simulink model "test_3"  (R2022b)
settings: Solver=VariableStepAuto  StartTime=0.0  StopTime=120  RelTol=1e-3
undefined symbols (not defined in the file): c, DenPlant, NumPlant
settings Model: Creator=JOWAKO  LastModifiedBy=JOWAKO

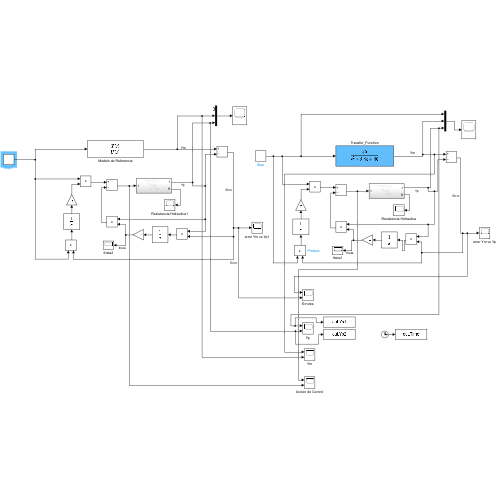
[thumbnail: Simulink's stored preview of the top-level diagram]
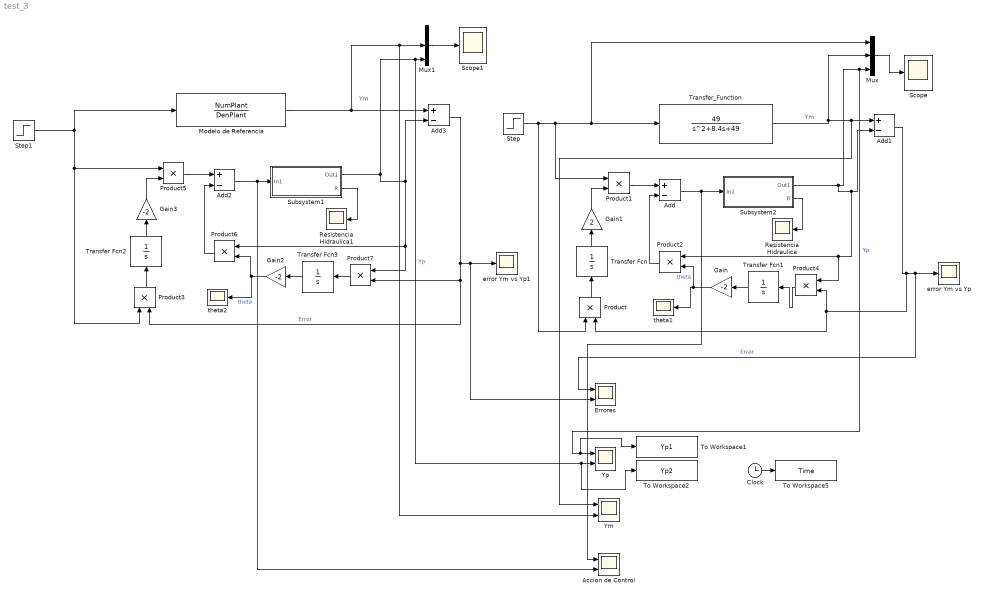
== system test_3 ==
  note: Ym
  note: Ym
  Accion de Control : Scope  NumInputPorts=2
  Add{,1..3} (4 alike) : Sum  Inputs=+-
  Clock : Clock
  Errores : Scope  NumInputPorts=2
  Gain : Gain  Gain=-2
  Gain1 : Gain  Gain=2
  Gain2 : Gain  Gain=-2
  Gain3 : Gain  Gain=-2
  Modelo de Referencia : TransferFcn  Numerator=NumPlant  Denominator=DenPlant
  Mux : Mux  Inputs=3
  Mux1 : Mux  Inputs=3
  Product{,1..7} (8 alike) : Product
  Resistencia Hidraulica : Scope
  Resistencia Hidraulica1 : Scope
  Scope : Scope
  Scope1 : Scope
  Step : Step  SampleTime=0
  Step1 : Step  SampleTime=0
  Subsystem1 : Subsystem
  Subsystem2 : Subsystem
  To Workspace1 : ToWorkspace  VariableName=Yp1  SaveFormat=Timeseries  SampleTime=-1
  To Workspace2 : ToWorkspace  VariableName=Yp2  SaveFormat=Timeseries  SampleTime=-1
  To Workspace5 : ToWorkspace  VariableName=Time  SaveFormat=Timeseries  SampleTime=-1
  Transfer Fcn{,1..3} (4 alike) : TransferFcn  Denominator=[1 0]
  Transfer_Function : TransferFcn  Numerator=49  Denominator=[1 8.4 49]
  Ym : Scope  NumInputPorts=2
  Yp : Scope  NumInputPorts=2
  error Ym vs Yp : Scope
  error Ym vs Yp1 : Scope
  theta1 : Scope
  theta2 : Scope
  wires:
  Subsystem2/2(R) -> Resistencia Hidraulica/1
  Transfer Fcn1/1 -> Gain/1
  Step1/1 -> Modelo de Referencia/1, Product5/1, Product3/1
  Transfer Fcn/1 -> Gain1/1
  Product2/1 -> Add/2
  Product1/1 -> Add/1
  Subsystem2/1(Out1) -> Add1/2, Product2/1, Product4/1, To Workspace1/1, Yp/1, Mux/3  "Yp"
  Add/1 -> Subsystem2/1(In1), Accion de Control/1
  Mux/1 -> Scope/1
  Gain1/1 -> Product1/2
  Transfer_Function/1 -> Mux/2, Ym/1, Add1/1
  Product/1 -> Transfer Fcn/1
  Add1/1 -> Errores/1, error Ym vs Yp/1, Product4/2, Product/2  "Error"
  Gain/1 -> theta1/1, Product2/2  "theta"
  Product4/1 -> Transfer Fcn1/1
  Subsystem1/2(R) -> Resistencia Hidraulica1/1
  Transfer Fcn3/1 -> Gain2/1
  Transfer Fcn2/1 -> Gain3/1
  Product6/1 -> Add2/2
  Product5/1 -> Add2/1
  Subsystem1/1(Out1) -> Add3/2, Product6/1, Product7/1, To Workspace2/1, Yp/2, Mux1/3  "Yp"
  Add2/1 -> Accion de Control/2, Subsystem1/1(In1)
  Mux1/1 -> Scope1/1
  Gain3/1 -> Product5/2
  Modelo de Referencia/1 -> Ym/2, Mux1/2, Add3/1
  Product3/1 -> Transfer Fcn2/1
  Add3/1 -> error Ym vs Yp1/1, Errores/2, Product3/2, Product7/2  "Error"
  Gain2/1 -> theta2/1, Product6/2  "theta"
  Product7/1 -> Transfer Fcn3/1
  Clock/1 -> To Workspace5/1
  Step/1 -> Product/1, Product1/1, Mux/1, Transfer_Function/1

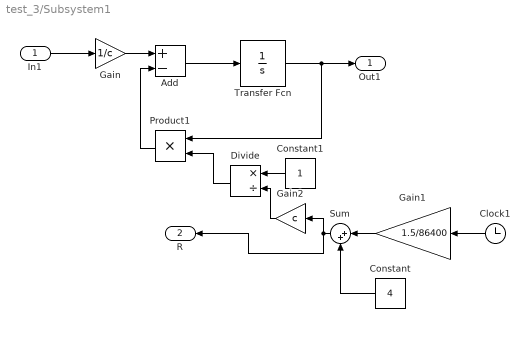
== system test_3/Subsystem1 ==
  In1 : Inport
  Add : Sum  Inputs=+-
  Clock1 : Clock
  Constant : Constant  Value=4
  Constant1 : Constant
  Divide : Product  Inputs=*/
  Gain : Gain  Gain=1/c
  Gain1 : Gain  Gain=1.5/86400
  Gain2 : Gain  Gain=c
  Product1 : Product
  Sum : Sum  Inputs=|++
  Transfer Fcn : TransferFcn  Denominator=[1 0]
  Out1 : Outport
  R : Outport  Port=2
  wires:
  In1/1 -> Gain/1
  Transfer Fcn/1 -> Product1/1, Out1/1
  Gain/1 -> Add/1
  Add/1 -> Transfer Fcn/1
  Clock1/1 -> Gain1/1
  Constant/1 -> Sum/2
  Gain1/1 -> Sum/1
  Product1/1 -> Add/2
  Sum/1 -> Gain2/1, R/1
  Constant1/1 -> Divide/1
  Divide/1 -> Product1/2
  Gain2/1 -> Divide/2

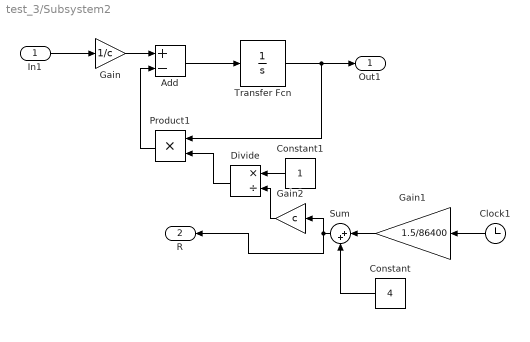
== system test_3/Subsystem2 ==
  In1 : Inport
  Add : Sum  Inputs=+-
  Clock1 : Clock
  Constant : Constant  Value=4
  Constant1 : Constant
  Divide : Product  Inputs=*/
  Gain : Gain  Gain=1/c
  Gain1 : Gain  Gain=1.5/86400
  Gain2 : Gain  Gain=c
  Product1 : Product
  Sum : Sum  Inputs=|++
  Transfer Fcn : TransferFcn  Denominator=[1 0]
  Out1 : Outport
  R : Outport  Port=2
  wires:
  In1/1 -> Gain/1
  Transfer Fcn/1 -> Product1/1, Out1/1
  Gain/1 -> Add/1
  Add/1 -> Transfer Fcn/1
  Clock1/1 -> Gain1/1
  Constant/1 -> Sum/2
  Gain1/1 -> Sum/1
  Product1/1 -> Add/2
  Sum/1 -> Gain2/1, R/1
  Constant1/1 -> Divide/1
  Divide/1 -> Product1/2
  Gain2/1 -> Divide/2
